simulink model "singlcontact_control_smc_lqr_mydimes_reaction"  (R2024a)
settings: Solver=VariableStepAuto  StartTime=0.0  StopTime=10  FixedStep=0.001  RelTol=1e-3
values from neighbouring files (symbols this model uses):
  ankle_servo_kd = 8    [robotParametersCtrl_mydiem_block_zmp.m]    (also in robotParametersCtrl_quad_modify_mydiem.m; robotParametersCtrl_quad_modify_mydiem_reaction.m)
  ankle_servo_ki = 4    [robotParametersCtrl_mydiem_block_zmp.m]    (also in robotParametersCtrl_quad_modify_mydiem.m; robotParametersCtrl_quad_modify_mydiem_reaction.m)
  ankle_servo_kp = 20    [robotParametersCtrl_mydiem_block_zmp.m]    (also in robotParametersCtrl_quad_modify_mydiem.m; robotParametersCtrl_quad_modify_mydiem_reaction.m)
  deriv_filter_coeff = 100    [robotParametersCtrl_mydiem_block_zmp.m]    (also in robotParametersCtrl_quad_modify_mydiem.m; robotParametersCtrl_quad_modify_mydiem_reaction.m)
  filter_coefficent_pid = 100    [robotParametersCtrl_mydiem_block_zmp.m]    (also in robotParametersCtrl_quad_modify_mydiem.m; robotParametersCtrl_quad_modify_mydiem_reaction.m)
  filter_coefficent_pids = 100    [robotParametersCtrl_quad_modify_mydiem_reaction.m]
  foot_z = 1.5    [robotParametersCtrl_mydiem_block_zmp.m]    (also in robotParametersCtrl_quad_modify_mydiem.m; robotParametersCtrl_quad_modify_mydiem_reaction.m)
  g = 9.81    [ABCDvalues_lqr_quad_mydime_reaction.m]    (also in robotParametersCtrl_mydiem_block_zmp.m = 9.80665; robotParametersCtrl_quad_modify_mydiem.m = 9.80665; robotParametersCtrl_quad_modify_mydiem_reaction.m = 9.80665)
  h = 32    [robotParametersCtrl_mydiem_block_zmp.m]    (also in robotParametersCtrl_quad_modify_mydiem.m; robotParametersCtrl_quad_modify_mydiem_reaction.m)
  height_plane = 0.025    [robotParametersCtrl_mydiem_block_zmp.m]    (also in robotParametersCtrl_quad_modify_mydiem.m; robotParametersCtrl_quad_modify_mydiem_reaction.m)
  hip_pitch_deriv = 20    [robotParametersCtrl_mydiem_block_zmp.m]    (also in robotParametersCtrl_quad_modify_mydiem.m = 200; robotParametersCtrl_quad_modify_mydiem_reaction.m = 200)
  hip_pitch_derivs = 200    [robotParametersCtrl_quad_modify_mydiem_reaction.m]
  hip_pitch_int = 0    [robotParametersCtrl_mydiem_block_zmp.m]    (also in robotParametersCtrl_quad_modify_mydiem.m = 150; robotParametersCtrl_quad_modify_mydiem_reaction.m = 150)
  hip_pitch_ints = 1500    [robotParametersCtrl_quad_modify_mydiem_reaction.m]
  hip_pitch_prop = 10    [robotParametersCtrl_mydiem_block_zmp.m]    (also in robotParametersCtrl_quad_modify_mydiem.m = 500; robotParametersCtrl_quad_modify_mydiem_reaction.m = 500)
  hip_pitch_props = 500    [robotParametersCtrl_quad_modify_mydiem_reaction.m]
  hip_roll_deriv = 28    [robotParametersCtrl_mydiem_block_zmp.m]    (also in robotParametersCtrl_quad_modify_mydiem.m = 280; robotParametersCtrl_quad_modify_mydiem_reaction.m = 280)
  hip_roll_derivs = 280    [robotParametersCtrl_quad_modify_mydiem_reaction.m]
  hip_roll_int = 0    [robotParametersCtrl_mydiem_block_zmp.m]    (also in robotParametersCtrl_quad_modify_mydiem.m = 180; robotParametersCtrl_quad_modify_mydiem_reaction.m = 180)
  hip_roll_ints = 180    [robotParametersCtrl_quad_modify_mydiem_reaction.m]
  hip_roll_prop = 10    [robotParametersCtrl_mydiem_block_zmp.m]    (also in robotParametersCtrl_quad_modify_mydiem.m = 300; robotParametersCtrl_quad_modify_mydiem_reaction.m = 300)
  hip_roll_props = 300    [robotParametersCtrl_quad_modify_mydiem_reaction.m]
  hip_servo_kd = 20    [robotParametersCtrl_mydiem_block_zmp.m]    (also in robotParametersCtrl_quad_modify_mydiem.m; robotParametersCtrl_quad_modify_mydiem_reaction.m)
  hip_servo_ki = 10    [robotParametersCtrl_mydiem_block_zmp.m]    (also in robotParametersCtrl_quad_modify_mydiem.m; robotParametersCtrl_quad_modify_mydiem_reaction.m)
  hip_servo_kp = 60    [robotParametersCtrl_mydiem_block_zmp.m]    (also in robotParametersCtrl_quad_modify_mydiem.m; robotParametersCtrl_quad_modify_mydiem_reaction.m)
  hip_smc_lamda = 85    [robotParametersCtrl_mydiem_block_zmp.m]    (also in robotParametersCtrl_quad_modify_mydiem.m; robotParametersCtrl_quad_modify_mydiem_reaction.m = 95)
  hip_smc_lamdas = 85    [robotParametersCtrl_quad_modify_mydiem_reaction.m]
  hip_smc_new = 25    [robotParametersCtrl_mydiem_block_zmp.m]    (also in robotParametersCtrl_quad_modify_mydiem.m; robotParametersCtrl_quad_modify_mydiem_reaction.m = 45)
  hip_smc_news = 25    [robotParametersCtrl_quad_modify_mydiem_reaction.m]
  init_angs_L = init_angs_R    [robotParametersCtrl_mydiem_block_zmp.m]    (also in robotParametersCtrl_quad_modify_mydiem.m; robotParametersCtrl_quad_modify_mydiem_reaction.m)
  init_angs_R = [0 -sum(init_angs) init_angs(2) 0 init_angs(1)]    [robotParametersCtrl_mydiem_block_zmp.m]    (also in robotParametersCtrl_quad_modify_mydiem.m; robotParametersCtrl_quad_modify_mydiem_reaction.m)
  init_height = h +                torso_z/2 + torso_offset_z + height_plane/2    (= 39.5125)    [robotParametersCtrl_mydiem_block_zmp.m]    (also in robotParametersCtrl_quad_modify_mydiem.m; robotParametersCtrl_quad_modify_mydiem_reaction.m)
  K = lqr(A, B, Q, R)    [ABCDvalues_lqr_quad_mydime_reaction.m]
  knee_pitch_deriv = 10    [robotParametersCtrl_mydiem_block_zmp.m]    (also in robotParametersCtrl_quad_modify_mydiem.m = 100; robotParametersCtrl_quad_modify_mydiem_reaction.m = 100)
  knee_pitch_derivs = 180    [robotParametersCtrl_quad_modify_mydiem_reaction.m]
  knee_pitch_int = 0    [robotParametersCtrl_mydiem_block_zmp.m]    (also in robotParametersCtrl_quad_modify_mydiem.m = 300; robotParametersCtrl_quad_modify_mydiem_reaction.m = 300)
  knee_pitch_ints = 7500    [robotParametersCtrl_quad_modify_mydiem_reaction.m]
  knee_pitch_prop = 10    [robotParametersCtrl_mydiem_block_zmp.m]    (also in robotParametersCtrl_quad_modify_mydiem.m = 400; robotParametersCtrl_quad_modify_mydiem_reaction.m = 400)
  knee_pitch_props = 1200    [robotParametersCtrl_quad_modify_mydiem_reaction.m]
  knee_servo_kd = 10    [robotParametersCtrl_mydiem_block_zmp.m]    (also in robotParametersCtrl_quad_modify_mydiem.m; robotParametersCtrl_quad_modify_mydiem_reaction.m)
  knee_servo_ki = 5    [robotParametersCtrl_mydiem_block_zmp.m]    (also in robotParametersCtrl_quad_modify_mydiem.m; robotParametersCtrl_quad_modify_mydiem_reaction.m)
  knee_servo_kp = 60    [robotParametersCtrl_mydiem_block_zmp.m]    (also in robotParametersCtrl_quad_modify_mydiem.m; robotParametersCtrl_quad_modify_mydiem_reaction.m)
  knee_smc_lamda = 140    [robotParametersCtrl_mydiem_block_zmp.m]    (also in robotParametersCtrl_quad_modify_mydiem.m; robotParametersCtrl_quad_modify_mydiem_reaction.m = 150)
  knee_smc_lamdas = 100    [robotParametersCtrl_quad_modify_mydiem_reaction.m]
  knee_smc_new = 80    [robotParametersCtrl_mydiem_block_zmp.m]    (also in robotParametersCtrl_quad_modify_mydiem.m; robotParametersCtrl_quad_modify_mydiem_reaction.m)
  knee_smc_news = 60    [robotParametersCtrl_quad_modify_mydiem_reaction.m]
  Kwalk = 0.6    [robotParametersCtrl_mydiem_block_zmp.m]    (also in robotParametersCtrl_quad_modify_mydiem.m; robotParametersCtrl_quad_modify_mydiem_reaction.m)
  l1 = 0.20    (= 0.2)    [ABCDvalues_lqr_quad_mydime_reaction.m]
  l2 = 0.20    (= 0.2)    [ABCDvalues_lqr_quad_mydime_reaction.m]
  lower_leg_length = 20    [robotParametersCtrl_mydiem_block_zmp.m]    (also in robotParametersCtrl_quad_modify_mydiem.m; robotParametersCtrl_quad_modify_mydiem_reaction.m)
  m1 = 0.45    [ABCDvalues_lqr_quad_mydime_reaction.m]
  m2 = 0.065    [ABCDvalues_lqr_quad_mydime_reaction.m]
  max_torque = 20    [robotParametersCtrl_mydiem_block_zmp.m]    (also in robotParametersCtrl_quad_modify_mydiem.m; robotParametersCtrl_quad_modify_mydiem_reaction.m)
  motion_time_constant = 0.01    [robotParametersCtrl_mydiem_block_zmp.m]    (also in robotParametersCtrl_quad_modify_mydiem.m; robotParametersCtrl_quad_modify_mydiem_reaction.m)
  plane_x = 25    [robotParametersCtrl_mydiem_block_zmp.m]    (also in robotParametersCtrl_quad_modify_mydiem.m; robotParametersCtrl_quad_modify_mydiem_reaction.m)
  plane_y = 3    [robotParametersCtrl_mydiem_block_zmp.m]    (also in robotParametersCtrl_quad_modify_mydiem.m; robotParametersCtrl_quad_modify_mydiem_reaction.m)
  stepHeight = 0.4    [ABCDvalues_lqr_quad_mydime_reaction.m]
  torso_offset_x = 17    [robotParametersCtrl_mydiem_block_zmp.m]    (also in robotParametersCtrl_quad_modify_mydiem.m; robotParametersCtrl_quad_modify_mydiem_reaction.m)
  torso_offset_x1 = -17    [robotParametersCtrl_mydiem_block_zmp.m]    (also in robotParametersCtrl_quad_modify_mydiem.m; robotParametersCtrl_quad_modify_mydiem_reaction.m)
  torso_offset_z = 0    [robotParametersCtrl_mydiem_block_zmp.m]    (also in robotParametersCtrl_quad_modify_mydiem.m; robotParametersCtrl_quad_modify_mydiem_reaction.m)
  torso_x = 40    [robotParametersCtrl_mydiem_block_zmp.m]    (also in robotParametersCtrl_quad_modify_mydiem.m; robotParametersCtrl_quad_modify_mydiem_reaction.m)
  torso_y = 20    [robotParametersCtrl_mydiem_block_zmp.m]    (also in robotParametersCtrl_quad_modify_mydiem.m; robotParametersCtrl_quad_modify_mydiem_reaction.m)
  torso_z = 15    [robotParametersCtrl_mydiem_block_zmp.m]    (also in robotParametersCtrl_quad_modify_mydiem.m; robotParametersCtrl_quad_modify_mydiem_reaction.m)
  Ts = 0.05    [ABCDvalues_lqr_quad_mydime_reaction.m]
  TsCtrl = 0.05    [robotParametersCtrl_mydiem_block_zmp.m]    (also in robotParametersCtrl_quad_modify_mydiem.m; robotParametersCtrl_quad_modify_mydiem_reaction.m)
  tWalk = 0.3    [robotParametersCtrl_mydiem_block_zmp.m]    (also in robotParametersCtrl_quad_modify_mydiem.m; robotParametersCtrl_quad_modify_mydiem_reaction.m)
  upper_leg_length = 20    [robotParametersCtrl_mydiem_block_zmp.m]    (also in robotParametersCtrl_quad_modify_mydiem.m; robotParametersCtrl_quad_modify_mydiem_reaction.m)
undefined symbols (not defined in the file or in its folder): X, Y, Z
libraries: simulink_extras x256, slpidlib x128, sm_lib x71, simulink x43, nesl_utility x35, walkingRobotUtils x21, dspsrcs4 x18, dspobslib x8
(part 23 of 33)

== system singlcontact_control_smc_lqr_mydimes_reaction/Walking Robot/smc+lqr/SMC Controllers FR2/SMC ==
  In1 : Inport
  In2 : Inport  Port=2
  T1_neuro : Inport  Port=3
  T2_neuro : Inport  Port=4
  Add : Sum
  Add1 : Sum
  Edot : Derivative
  Edot1 : Derivative
  Gain : Gain  Gain=-0.9
  Gain1 : Gain  Gain=-0.9
  Mux : Mux  Inputs=2
  New : Gain  Gain=knee_smc_new
  New1 : Gain  Gain=hip_smc_new
  Product : Product
  Product2 : Product
  S : Sum
  S1 : Sum
  Scope : Scope  NumInputPorts=2
  Scope{2..5} (4 alike) : Scope
  Sum : Sum  Inputs=++++
  Sum1 : Sum  Inputs=++++
  Tanh : Trigonometry  Operator=tanh
  Tanh1 : Trigonometry  Operator=tanh
  lamda : Constant  Value=knee_smc_lamda
  lamda1 : Constant  Value=hip_smc_lamda
  Out1 : Outport
  tag scope: edotBR1=global, edotBR2=global, lamdaBR1=global, lamdaBR2=global
  wires:
  S1/1 -> Tanh/1
  Edot/1 -> [edotBR1], S/1
  Product/1 -> S/2
  lamda1/1 -> [lamdaBR2], Product2/1
  In2/1 -> Product2/2, Edot1/1
  New1/1 -> Add1/1, Sum1/1
  Product2/1 -> S1/2
  In1/1 -> Edot/1, Product/2
  Edot1/1 -> S1/1, [edotBR2]
  Tanh1/1 -> New/1
  lamda/1 -> [lamdaBR1], Product/1
  Tanh/1 -> New1/1
  New/1 -> Sum/1, Add/1, Scope/1
  [TT1BR] -> Scope/2, Add/2, Sum/2
  [TT2BR] -> Add1/2, Sum1/2
  Mux/1 -> Out1/1
  Sum/1 -> Scope3/1, Scope5/1, Mux/1
  Sum1/1 -> Scope4/1, Mux/2, Scope2/1
  T1_neuro/1 -> Sum/3
  T2_neuro/1 -> Sum1/3
  S/1 -> Tanh1/1
  Add/1 -> Gain/1
  Gain/1 -> ?
  Gain1/1 -> ?
  Add1/1 -> Gain1/1

== system singlcontact_control_smc_lqr_mydimes_reaction/Walking Robot/smc+lqr/SMC Controllers FR3/Equivalent control ==
  theta2 : Inport
  theta1 : Inport  Port=2
  theta2ddot : Inport  Port=3
  theta1dot : Inport  Port=4
  theta2dot : Inport  Port=5
  theta1ddot : Inport  Port=6
  theta3 : Inport  Port=7
  theta4 : Inport  Port=8
  theta1dot1 : Inport  Port=9
  Constant : Constant  Value=0
  Constant1 : Constant  Value=0
  SMC equivalent T1 : Subsystem
  SMC equivalent T2 : Subsystem
  Scope : Scope  NumInputPorts=2
  tag scope: TT1BL=global, TT2BL=global
  wires:
  theta1dot1/1 -> SMC equivalent T2/5(theta1dot)
  theta2dot/1 -> SMC equivalent T1/5(theta2dot)
  theta1ddot/1 -> SMC equivalent T2/1(theta1ddot)
  theta4/1 -> SMC equivalent T2/3(theta1)
  theta1/1 -> SMC equivalent T1/2(theta1)
  theta3/1 -> SMC equivalent T2/2(theta2)
  Constant/1 -> SMC equivalent T1/6(theta1ddot)
  theta1dot/1 -> SMC equivalent T1/4(theta1dot)
  theta2ddot/1 -> SMC equivalent T1/3(theta2ddot)
  Constant1/1 -> SMC equivalent T2/4(theta2ddot)
  SMC equivalent T1/1(T1) -> [TT1BL], Scope/2
  theta2/1 -> SMC equivalent T1/1(theta2)
  SMC equivalent T2/1(T2) -> [TT2BL], Scope/1

== system singlcontact_control_smc_lqr_mydimes_reaction/Walking Robot/smc+lqr/SMC Controllers FR3/SMC ==
  In1 : Inport
  In2 : Inport  Port=2
  T1_neuro : Inport  Port=3
  T2_neuro : Inport  Port=4
  Add : Sum
  Add1 : Sum
  Edot : Derivative
  Edot1 : Derivative
  Gain : Gain  Gain=-0.9
  Gain1 : Gain  Gain=-0.9
  Mux : Mux  Inputs=2
  New : Gain  Gain=knee_smc_new
  New1 : Gain  Gain=hip_smc_new
  Product : Product
  Product2 : Product
  S : Sum
  S1 : Sum
  Scope : Scope  NumInputPorts=2
  Scope{2..5} (4 alike) : Scope
  Sum : Sum  Inputs=++++
  Sum1 : Sum  Inputs=++++
  Tanh : Trigonometry  Operator=tanh
  Tanh1 : Trigonometry  Operator=tanh
  lamda : Constant  Value=knee_smc_lamda
  lamda1 : Constant  Value=hip_smc_lamda
  Out1 : Outport
  tag scope: edotBL1=global, edotBL2=global, lamdaBL1=global, lamdaBL2=global
  wires:
  Add1/1 -> Gain1/1
  Gain1/1 -> ?
  Gain/1 -> ?
  Add/1 -> Gain/1
  S/1 -> Tanh1/1
  T2_neuro/1 -> Sum1/3
  T1_neuro/1 -> Sum/3
  Sum1/1 -> Scope2/1, Mux/2, Scope4/1
  Sum/1 -> Mux/1, Scope5/1, Scope3/1
  Mux/1 -> Out1/1
  [TT2BL] -> Sum1/2, Add1/2
  [TT1BL] -> Sum/2, Add/2, Scope/2
  New/1 -> Scope/1, Add/1, Sum/1
  Tanh/1 -> New1/1
  lamda/1 -> Product/1, [lamdaBL1]
  Tanh1/1 -> New/1
  Edot1/1 -> [edotBL2], S1/1
  In1/1 -> Product/2, Edot/1
  Product2/1 -> S1/2
  New1/1 -> Sum1/1, Add1/1
  In2/1 -> Edot1/1, Product2/2
  lamda1/1 -> Product2/1, [lamdaBL2]
  Product/1 -> S/2
  Edot/1 -> S/1, [edotBL1]
  S1/1 -> Tanh/1

== system singlcontact_control_smc_lqr_mydimes_reaction/Walking Robot/smc+lqr/SMC Controllers FR4/Equivalent control ==
  theta2 : Inport
  theta1 : Inport  Port=2
  theta2ddot : Inport  Port=3
  theta1dot : Inport  Port=4
  theta2dot : Inport  Port=5
  theta1ddot : Inport  Port=6
  theta3 : Inport  Port=7
  theta4 : Inport  Port=8
  theta1dot1 : Inport  Port=9
  Constant : Constant  Value=0
  Constant1 : Constant  Value=0
  SMC equivalent T1 : Subsystem
  SMC equivalent T2 : Subsystem
  Scope : Scope  NumInputPorts=2
  tag scope: TT1FR=global, TT2FR=global
  wires:
  SMC equivalent T2/1(T2) -> Scope/1, [TT2FR]
  theta2/1 -> SMC equivalent T1/1(theta2)
  SMC equivalent T1/1(T1) -> Scope/2, [TT1FR]
  Constant1/1 -> SMC equivalent T2/4(theta2ddot)
  theta2ddot/1 -> SMC equivalent T1/3(theta2ddot)
  theta1dot/1 -> SMC equivalent T1/4(theta1dot)
  Constant/1 -> SMC equivalent T1/6(theta1ddot)
  theta3/1 -> SMC equivalent T2/2(theta2)
  theta1/1 -> SMC equivalent T1/2(theta1)
  theta4/1 -> SMC equivalent T2/3(theta1)
  theta1ddot/1 -> SMC equivalent T2/1(theta1ddot)
  theta2dot/1 -> SMC equivalent T1/5(theta2dot)
  theta1dot1/1 -> SMC equivalent T2/5(theta1dot)

== system singlcontact_control_smc_lqr_mydimes_reaction/Walking Robot/smc+lqr/SMC Controllers FR4/SMC ==
  In1 : Inport
  In2 : Inport  Port=2
  T1_neuro : Inport  Port=3
  T2_neuro : Inport  Port=4
  Add : Sum
  Add1 : Sum
  Edot : Derivative
  Edot1 : Derivative
  Gain : Gain  Gain=-0.9
  Gain1 : Gain  Gain=-0.9
  Mux : Mux  Inputs=2
  New : Gain  Gain=knee_smc_new
  New1 : Gain  Gain=hip_smc_new
  Product : Product
  Product2 : Product
  S : Sum
  S1 : Sum
  Scope : Scope  NumInputPorts=2
  Scope{2..5} (4 alike) : Scope
  Sum : Sum  Inputs=++++
  Sum1 : Sum  Inputs=++++
  Tanh : Trigonometry  Operator=tanh
  Tanh1 : Trigonometry  Operator=tanh
  lamda : Constant  Value=knee_smc_lamda
  lamda1 : Constant  Value=hip_smc_lamda
  Out1 : Outport
  tag scope: edotFR1=global, edotFR2=global, lamdaFR1=global, lamdaFR2=global
  wires:
  S1/1 -> Tanh/1
  Edot/1 -> [edotFR1], S/1
  Product/1 -> S/2
  lamda1/1 -> [lamdaFR2], Product2/1
  In2/1 -> Product2/2, Edot1/1
  New1/1 -> Add1/1, Sum1/1
  Product2/1 -> S1/2
  In1/1 -> Edot/1, Product/2
  Edot1/1 -> S1/1, [edotFR2]
  Tanh1/1 -> New/1
  lamda/1 -> [lamdaFR1], Product/1
  Tanh/1 -> New1/1
  New/1 -> Sum/1, Add/1, Scope/1
  [TT1FR] -> Scope/2, Add/2, Sum/2
  [TT2FR] -> Add1/2, Sum1/2
  Mux/1 -> Out1/1
  Sum/1 -> Scope3/1, Scope5/1, Mux/1
  Sum1/1 -> Scope4/1, Mux/2, Scope2/1
  T1_neuro/1 -> Sum/3
  T2_neuro/1 -> Sum1/3
  S/1 -> Tanh1/1
  Add/1 -> Gain/1
  Gain/1 -> ?
  Gain1/1 -> ?
  Add1/1 -> Gain1/1

== system singlcontact_control_smc_lqr_mydimes_reaction/Walking Robot/smc+lqr+neuro1+reaction1/SMC Controllers BL/Equivalent control ==
  theta2 : Inport
  theta1 : Inport  Port=2
  theta2ddot : Inport  Port=3
  theta1dot : Inport  Port=4
  theta2dot : Inport  Port=5
  theta1ddot : Inport  Port=6
  theta3 : Inport  Port=7
  theta4 : Inport  Port=8
  theta1dot1 : Inport  Port=9
  Constant : Constant  Value=0
  Constant1 : Constant  Value=0
  SMC equivalent T1 : Subsystem
  SMC equivalent T2 : Subsystem
  Scope : Scope  NumInputPorts=2
  tag scope: TT1BL=global, TT2BL=global
  wires:
  theta1dot1/1 -> SMC equivalent T2/5(theta1dot)
  theta2dot/1 -> SMC equivalent T1/5(theta2dot)
  theta1ddot/1 -> SMC equivalent T2/1(theta1ddot)
  theta4/1 -> SMC equivalent T2/3(theta1)
  theta1/1 -> SMC equivalent T1/2(theta1)
  theta3/1 -> SMC equivalent T2/2(theta2)
  Constant/1 -> SMC equivalent T1/6(theta1ddot)
  theta1dot/1 -> SMC equivalent T1/4(theta1dot)
  theta2ddot/1 -> SMC equivalent T1/3(theta2ddot)
  Constant1/1 -> SMC equivalent T2/4(theta2ddot)
  SMC equivalent T1/1(T1) -> [TT1BL], Scope/2
  theta2/1 -> SMC equivalent T1/1(theta2)
  SMC equivalent T2/1(T2) -> [TT2BL], Scope/1

== system singlcontact_control_smc_lqr_mydimes_reaction/Walking Robot/smc+lqr+neuro1+reaction1/SMC Controllers BL/SMC ==
  In1 : Inport
  In2 : Inport  Port=2
  T1_neuro : Inport  Port=3
  T2_neuro : Inport  Port=4
  Input : Inport  Port=5
  Input1 : Inport  Port=6
  Edot : Derivative
  Edot1 : Derivative
  Gain : Gain  Gain=-0.85
  Gain1 : Gain  Gain=-0.7
  Mux : Mux  Inputs=2
  New : Gain  Gain=knee_smc_new
  New1 : Gain  Gain=hip_smc_new
  Product : Product
  Product2 : Product
  Random Source1 : dspobslib/Random Source  SrcType=Uniform  NormMethod=Ziggurat  CltLength=12  MinVal=-1  MaxVal=1  MeanVal=0  VarVal=1  RepMode=Not repeatable  rawSeed=1  IsInherit=off  SampMode=Discrete  SampTime=0.005  SampFrame=1  DataType=Double  OutComplex=Real  OutputFrames=off
  Random Source2 : dspobslib/Random Source  SrcType=Uniform  NormMethod=Ziggurat  CltLength=12  MinVal=-1  MaxVal=1  MeanVal=0  VarVal=1  RepMode=Not repeatable  rawSeed=1  IsInherit=off  SampMode=Discrete  SampTime=0.005  SampFrame=1  DataType=Double  OutComplex=Real  OutputFrames=off
  S : Sum
  S1 : Sum
  Scope : Scope  NumInputPorts=2
  Scope{2..5} (4 alike) : Scope
  Sum : Sum  Inputs=+++++
  Sum1 : Sum  Inputs=+++++
  Tanh : Trigonometry  Operator=tanh
  Tanh1 : Trigonometry  Operator=tanh
  lamda : Constant  Value=knee_smc_lamda
  lamda1 : Constant  Value=hip_smc_lamda
  Out1 : Outport
  tag scope: edotBL1=global, edotBL2=global, lamdaBL1=global, lamdaBL2=global, slBL1=global, slBL2=global
  wires:
  New1/1 -> Sum1/1, Gain1/1
  Gain1/1 -> Sum1/4
  Gain/1 -> Sum/4
  New/1 -> Sum/1, Gain/1
  S/1 -> Tanh1/1, [slBL1]
  T2_neuro/1 -> Sum1/3
  T1_neuro/1 -> Sum/3
  Sum1/1 -> Scope2/1, Mux/2, Scope4/1
  Sum/1 -> Mux/1, Scope5/1, Scope3/1
  Mux/1 -> Out1/1
  [TT2BL] -> Sum1/2
  [TT1BL] -> Sum/2
  Tanh/1 -> New1/1
  lamda/1 -> Product/1, [lamdaBL1]
  Tanh1/1 -> New/1
  Edot1/1 -> [edotBL2], S1/1
  In1/1 -> Product/2, Edot/1
  Product2/1 -> S1/2
  In2/1 -> Edot1/1, Product2/2
  lamda1/1 -> Product2/1, [lamdaBL2]
  Product/1 -> S/2
  Edot/1 -> S/1, [edotBL1]
  S1/1 -> Tanh/1, [slBL2]
  Random Source1/1 -> ?
  Random Source2/1 -> ?
  Input/1 -> Sum/5
  Input1/1 -> Sum1/5

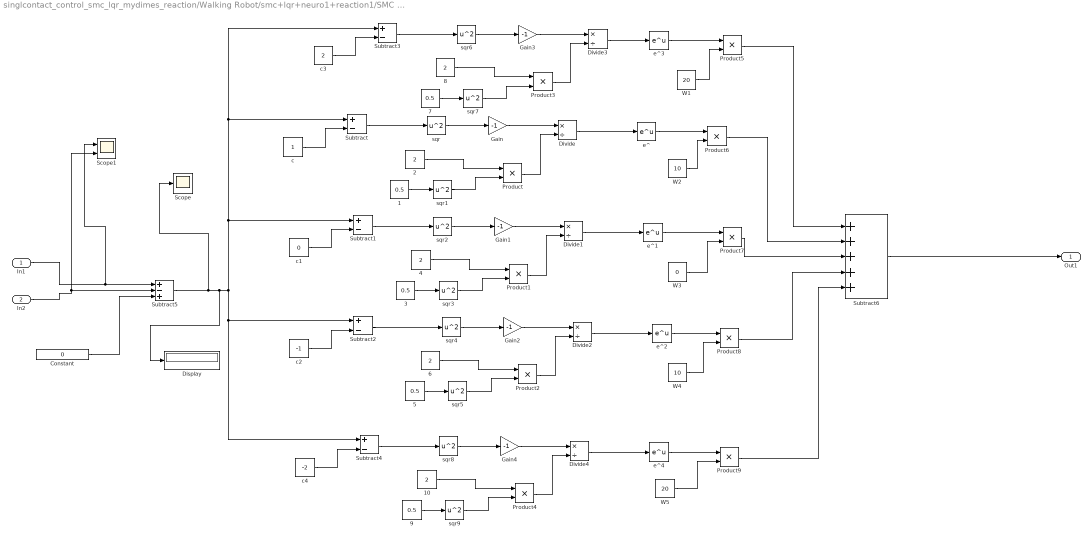
== system singlcontact_control_smc_lqr_mydimes_reaction/Walking Robot/smc+lqr+neuro1+reaction1/SMC Controllers BL/Subsystem ==
  In1 : Inport
  In2 : Inport  Port=2
  {1,3,5,7,9} (5 alike) : Constant  Value=0.5
  {2,4,6,8,10} (5 alike) : Constant  Value=2
  Constant : Constant  Value=0
  Display : Display
  Divide{,1..4} (5 alike) : Product  Inputs=*/
  Gain{,1..4} (5 alike) : Gain  Gain=-1
  Product{,1..9} (10 alike) : Product
  Scope : Scope
  Scope1 : Scope  NumInputPorts=2
  Subtract{,1..4} (5 alike) : Sum  Inputs=+-
  Subtract5 : Sum  Inputs=+-+
  Subtract6 : Sum  Inputs=+++++
  W1 : Constant  Value=20
  W2 : Constant  Value=10
  W3 : Constant  Value=0
  W4 : Constant  Value=10
  W5 : Constant  Value=20
  c : Constant
  c1 : Constant  Value=0
  c2 : Constant  Value=-1
  c3 : Constant  Value=2
  c4 : Constant  Value=-2
  e^{,1..4} (5 alike) : Math
  sqr{,1..9} (10 alike) : Math  Operator=square
  Out1 : Outport
  wires:
  Constant/1 -> Subtract5/3
  Divide3/1 -> e^3/1
  9/1 -> sqr9/1
  Product8/1 -> Subtract6/4
  Product7/1 -> Subtract6/3
  W4/1 -> Product8/2
  c2/1 -> Subtract2/2
  Product4/1 -> Divide4/2
  10/1 -> Product4/1
  e^3/1 -> Product5/1
  sqr6/1 -> Gain3/1
  6/1 -> Product2/1
  sqr3/1 -> Product1/2
  e^2/1 -> Product8/1
  Divide2/1 -> e^2/1
  Subtract2/1 -> sqr4/1
  Subtract6/1 -> Out1/1
  8/1 -> Product3/1
  sqr7/1 -> Product3/2
  Divide/1 -> e^/1
  5/1 -> sqr5/1
  3/1 -> sqr3/1
  4/1 -> Product1/1
  Gain2/1 -> Divide2/1
  Gain4/1 -> Divide4/1
  In1/1 -> Subtract5/1, Scope1/1
  W1/1 -> Product5/2
  sqr4/1 -> Gain2/1
  c3/1 -> Subtract3/2
  e^4/1 -> Product9/1
  sqr5/1 -> Product2/2
  sqr8/1 -> Gain4/1
  1/1 -> sqr1/1
  2/1 -> Product/1
  Product5/1 -> Subtract6/1
  Divide4/1 -> e^4/1
  W5/1 -> Product9/2
  7/1 -> sqr7/1
  Subtract/1 -> sqr/1
  Subtract5/1 -> Subtract2/1, Subtract4/1, Subtract3/1, Subtract/1, Subtract1/1, Display/1, Scope/1
  c1/1 -> Subtract1/2
  Subtract1/1 -> sqr2/1
  e^1/1 -> Product7/1
  Product9/1 -> Subtract6/5
  c4/1 -> Subtract4/2
  Subtract3/1 -> sqr6/1
  e^/1 -> Product6/1
  Product3/1 -> Divide3/2
  W2/1 -> Product6/2
  W3/1 -> Product7/2
  Gain1/1 -> Divide1/1
  Product6/1 -> Subtract6/2
  Product2/1 -> Divide2/2
  Gain/1 -> Divide/1
  Subtract4/1 -> sqr8/1
  Divide1/1 -> e^1/1
  Gain3/1 -> Divide3/1
  In2/1 -> Scope1/2, Subtract5/2
  sqr1/1 -> Product/2
  sqr2/1 -> Gain1/1
  Product/1 -> Divide/2
  sqr/1 -> Gain/1
  Product1/1 -> Divide1/2
  sqr9/1 -> Product4/2
  c/1 -> Subtract/2

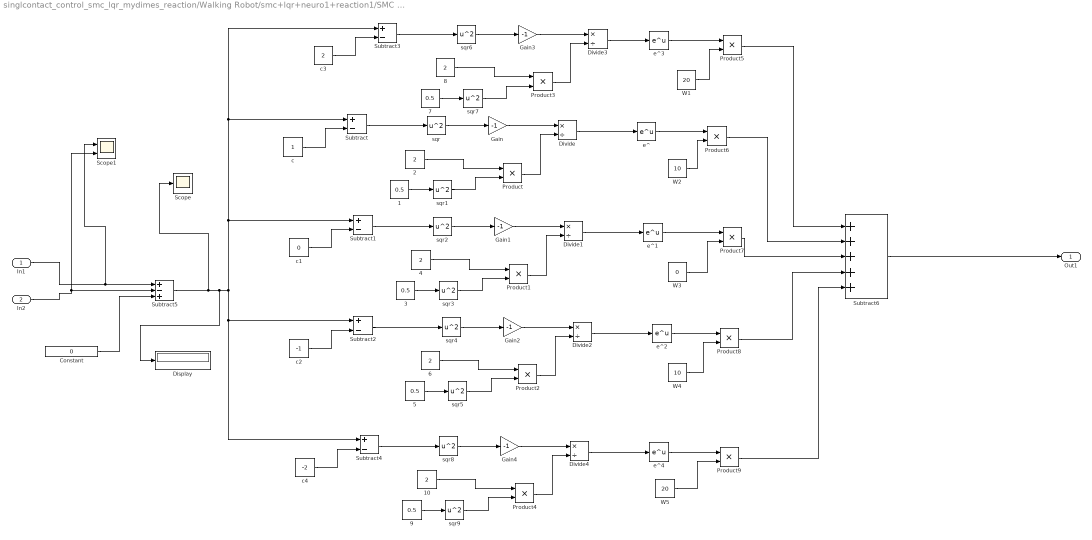
== system singlcontact_control_smc_lqr_mydimes_reaction/Walking Robot/smc+lqr+neuro1+reaction1/SMC Controllers BL/Subsystem1 ==
  In1 : Inport
  In2 : Inport  Port=2
  {1,3,5,7,9} (5 alike) : Constant  Value=0.5
  {2,4,6,8,10} (5 alike) : Constant  Value=2
  Constant : Constant  Value=0
  Display : Display
  Divide{,1..4} (5 alike) : Product  Inputs=*/
  Gain{,1..4} (5 alike) : Gain  Gain=-1
  Product{,1..9} (10 alike) : Product
  Scope : Scope
  Scope1 : Scope  NumInputPorts=2
  Subtract{,1..4} (5 alike) : Sum  Inputs=+-
  Subtract5 : Sum  Inputs=+-+
  Subtract6 : Sum  Inputs=+++++
  W1 : Constant  Value=20
  W2 : Constant  Value=10
  W3 : Constant  Value=0
  W4 : Constant  Value=10
  W5 : Constant  Value=20
  c : Constant
  c1 : Constant  Value=0
  c2 : Constant  Value=-1
  c3 : Constant  Value=2
  c4 : Constant  Value=-2
  e^{,1..4} (5 alike) : Math
  sqr{,1..9} (10 alike) : Math  Operator=square
  Out1 : Outport
  wires:
  c/1 -> Subtract/2
  sqr9/1 -> Product4/2
  Product1/1 -> Divide1/2
  sqr/1 -> Gain/1
  Product/1 -> Divide/2
  sqr2/1 -> Gain1/1
  sqr1/1 -> Product/2
  In2/1 -> Subtract5/2, Scope1/2
  Gain3/1 -> Divide3/1
  Divide1/1 -> e^1/1
  Subtract4/1 -> sqr8/1
  Gain/1 -> Divide/1
  Product2/1 -> Divide2/2
  Product6/1 -> Subtract6/2
  Gain1/1 -> Divide1/1
  W3/1 -> Product7/2
  W2/1 -> Product6/2
  Product3/1 -> Divide3/2
  e^/1 -> Product6/1
  Subtract3/1 -> sqr6/1
  c4/1 -> Subtract4/2
  Product9/1 -> Subtract6/5
  e^1/1 -> Product7/1
  Subtract1/1 -> sqr2/1
  c1/1 -> Subtract1/2
  Subtract5/1 -> Scope/1, Display/1, Subtract1/1, Subtract/1, Subtract3/1, Subtract4/1, Subtract2/1
  Subtract/1 -> sqr/1
  7/1 -> sqr7/1
  W5/1 -> Product9/2
  Divide4/1 -> e^4/1
  Product5/1 -> Subtract6/1
  2/1 -> Product/1
  1/1 -> sqr1/1
  sqr8/1 -> Gain4/1
  sqr5/1 -> Product2/2
  e^4/1 -> Product9/1
  c3/1 -> Subtract3/2
  sqr4/1 -> Gain2/1
  W1/1 -> Product5/2
  In1/1 -> Scope1/1, Subtract5/1
  Gain4/1 -> Divide4/1
  Gain2/1 -> Divide2/1
  4/1 -> Product1/1
  3/1 -> sqr3/1
  5/1 -> sqr5/1
  Divide/1 -> e^/1
  sqr7/1 -> Product3/2
  8/1 -> Product3/1
  Subtract6/1 -> Out1/1
  Subtract2/1 -> sqr4/1
  Divide2/1 -> e^2/1
  e^2/1 -> Product8/1
  sqr3/1 -> Product1/2
  6/1 -> Product2/1
  sqr6/1 -> Gain3/1
  e^3/1 -> Product5/1
  10/1 -> Product4/1
  Product4/1 -> Divide4/2
  c2/1 -> Subtract2/2
  W4/1 -> Product8/2
  Product7/1 -> Subtract6/3
  Product8/1 -> Subtract6/4
  9/1 -> sqr9/1
  Divide3/1 -> e^3/1
  Constant/1 -> Subtract5/3

== system singlcontact_control_smc_lqr_mydimes_reaction/Walking Robot/smc+lqr+neuro1+reaction1/SMC Controllers BL/Subsystem2 ==
  <knee_angle> : Inport
  <hip_pitch_angle> : Inport  Port=2
  Gain3 : Gain  Gain=0.5
  Product : Product
  Product3 : Product
  length from ground : Subsystem
  Input : Outport
  Input1 : Outport  Port=2
  wires:
  Product/1 -> Input/1
  length from ground/2(Outport) -> Product3/1
  Gain3/1 -> Product/2, Product3/2
  Product3/1 -> Input1/1
  [Rbl] -> Gain3/1
  <hip_pitch_angle>/1 -> length from ground/2(In2)
  <knee_angle>/1 -> length from ground/1(In1)
  length from ground/1(Output) -> Product/1

== system singlcontact_control_smc_lqr_mydimes_reaction/Walking Robot/smc+lqr+neuro1+reaction1/SMC Controllers BR/Equivalent control ==
  theta2 : Inport
  theta1 : Inport  Port=2
  theta2ddot : Inport  Port=3
  theta1dot : Inport  Port=4
  theta2dot : Inport  Port=5
  theta1ddot : Inport  Port=6
  theta3 : Inport  Port=7
  theta4 : Inport  Port=8
  theta1dot1 : Inport  Port=9
  Constant : Constant  Value=0
  Constant1 : Constant  Value=0
  SMC equivalent T1 : Subsystem
  SMC equivalent T2 : Subsystem
  Scope : Scope  NumInputPorts=2
  tag scope: TT1BR=global, TT2BR=global
  wires:
  SMC equivalent T2/1(T2) -> Scope/1, [TT2BR]
  theta2/1 -> SMC equivalent T1/1(theta2)
  SMC equivalent T1/1(T1) -> Scope/2, [TT1BR]
  Constant1/1 -> SMC equivalent T2/4(theta2ddot)
  theta2ddot/1 -> SMC equivalent T1/3(theta2ddot)
  theta1dot/1 -> SMC equivalent T1/4(theta1dot)
  Constant/1 -> SMC equivalent T1/6(theta1ddot)
  theta3/1 -> SMC equivalent T2/2(theta2)
  theta1/1 -> SMC equivalent T1/2(theta1)
  theta4/1 -> SMC equivalent T2/3(theta1)
  theta1ddot/1 -> SMC equivalent T2/1(theta1ddot)
  theta2dot/1 -> SMC equivalent T1/5(theta2dot)
  theta1dot1/1 -> SMC equivalent T2/5(theta1dot)

== system singlcontact_control_smc_lqr_mydimes_reaction/Walking Robot/smc+lqr+neuro1+reaction1/SMC Controllers BR/SMC ==
  In1 : Inport
  In2 : Inport  Port=2
  T1_neuro : Inport  Port=3
  T2_neuro : Inport  Port=4
  Input : Inport  Port=5
  Input1 : Inport  Port=6
  Edot : Derivative
  Edot1 : Derivative
  Gain : Gain  Gain=-0.85
  Gain1 : Gain  Gain=-0.7
  Mux : Mux  Inputs=2
  New : Gain  Gain=knee_smc_new
  New1 : Gain  Gain=hip_smc_new
  Product : Product
  Product2 : Product
  Random Source1 : dspobslib/Random Source  SrcType=Uniform  NormMethod=Ziggurat  CltLength=12  MinVal=-1  MaxVal=1  MeanVal=0  VarVal=1  RepMode=Not repeatable  rawSeed=1  IsInherit=off  SampMode=Discrete  SampTime=0.005  SampFrame=1  DataType=Double  OutComplex=Real  OutputFrames=off
  Random Source2 : dspobslib/Random Source  SrcType=Uniform  NormMethod=Ziggurat  CltLength=12  MinVal=-1  MaxVal=1  MeanVal=0  VarVal=1  RepMode=Not repeatable  rawSeed=1  IsInherit=off  SampMode=Discrete  SampTime=0.005  SampFrame=1  DataType=Double  OutComplex=Real  OutputFrames=off
  S : Sum
  S1 : Sum
  Scope : Scope  NumInputPorts=2
  Scope{2..5} (4 alike) : Scope
  Sum : Sum  Inputs=+++++
  Sum1 : Sum  Inputs=+++++
  Tanh : Trigonometry  Operator=tanh
  Tanh1 : Trigonometry  Operator=tanh
  lamda : Constant  Value=knee_smc_lamda
  lamda1 : Constant  Value=hip_smc_lamda
  Out1 : Outport
  tag scope: edotBR1=global, edotBR2=global, lamdaBR1=global, lamdaBR2=global, slBR1=global, slBR2=global
  wires:
  S1/1 -> [slBR2], Tanh/1
  Edot/1 -> [edotBR1], S/1
  Product/1 -> S/2
  lamda1/1 -> Product2/1, [lamdaBR2]
  In2/1 -> Product2/2, Edot1/1
  Product2/1 -> S1/2
  In1/1 -> Edot/1, Product/2
  Edot1/1 -> S1/1, [edotBR2]
  Tanh1/1 -> New/1
  lamda/1 -> [lamdaBR1], Product/1
  Tanh/1 -> New1/1
  [TT1BR] -> Sum/2
  [TT2BR] -> Sum1/2
  Mux/1 -> Out1/1
  Sum/1 -> Mux/1, Scope5/1, Scope3/1
  Sum1/1 -> Scope4/1, Mux/2, Scope2/1
  T1_neuro/1 -> Sum/3
  T2_neuro/1 -> Sum1/3
  S/1 -> [slBR1], Tanh1/1
  New/1 -> Gain/1, Sum/1
  Gain/1 -> Sum/4
  Gain1/1 -> Sum1/4
  New1/1 -> Sum1/1, Gain1/1
  Random Source1/1 -> ?
  Random Source2/1 -> ?
  Input/1 -> Sum/5
  Input1/1 -> Sum1/5

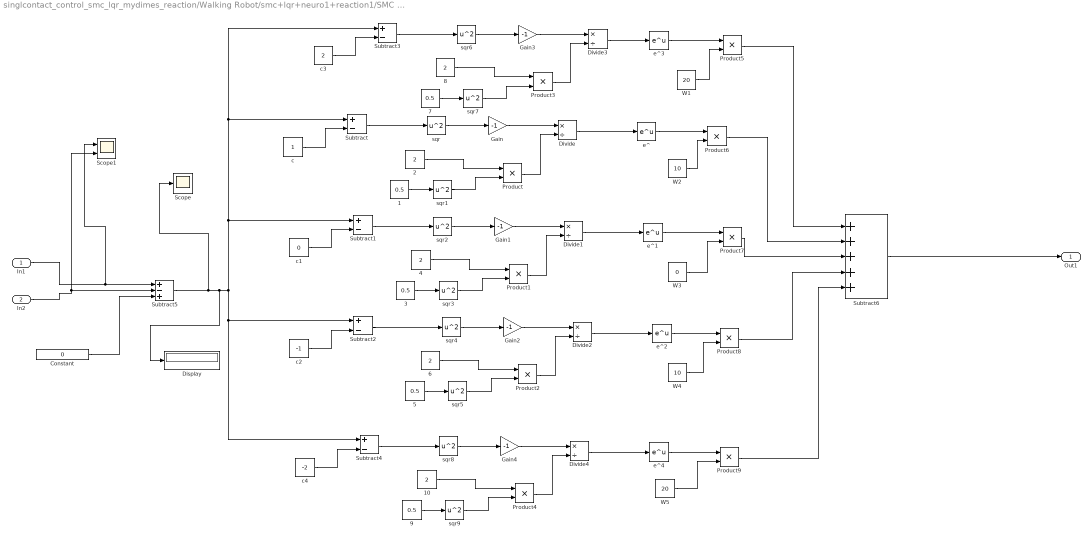
== system singlcontact_control_smc_lqr_mydimes_reaction/Walking Robot/smc+lqr+neuro1+reaction1/SMC Controllers BR/Subsystem ==
  In1 : Inport
  In2 : Inport  Port=2
  {1,3,5,7,9} (5 alike) : Constant  Value=0.5
  {2,4,6,8,10} (5 alike) : Constant  Value=2
  Constant : Constant  Value=0
  Display : Display
  Divide{,1..4} (5 alike) : Product  Inputs=*/
  Gain{,1..4} (5 alike) : Gain  Gain=-1
  Product{,1..9} (10 alike) : Product
  Scope : Scope
  Scope1 : Scope  NumInputPorts=2
  Subtract{,1..4} (5 alike) : Sum  Inputs=+-
  Subtract5 : Sum  Inputs=+-+
  Subtract6 : Sum  Inputs=+++++
  W1 : Constant  Value=20
  W2 : Constant  Value=10
  W3 : Constant  Value=0
  W4 : Constant  Value=10
  W5 : Constant  Value=20
  c : Constant
  c1 : Constant  Value=0
  c2 : Constant  Value=-1
  c3 : Constant  Value=2
  c4 : Constant  Value=-2
  e^{,1..4} (5 alike) : Math
  sqr{,1..9} (10 alike) : Math  Operator=square
  Out1 : Outport
  wires:
  c/1 -> Subtract/2
  sqr9/1 -> Product4/2
  Product1/1 -> Divide1/2
  sqr/1 -> Gain/1
  Product/1 -> Divide/2
  sqr2/1 -> Gain1/1
  sqr1/1 -> Product/2
  In2/1 -> Subtract5/2, Scope1/2
  Gain3/1 -> Divide3/1
  Divide1/1 -> e^1/1
  Subtract4/1 -> sqr8/1
  Gain/1 -> Divide/1
  Product2/1 -> Divide2/2
  Product6/1 -> Subtract6/2
  Gain1/1 -> Divide1/1
  W3/1 -> Product7/2
  W2/1 -> Product6/2
  Product3/1 -> Divide3/2
  e^/1 -> Product6/1
  Subtract3/1 -> sqr6/1
  c4/1 -> Subtract4/2
  Product9/1 -> Subtract6/5
  e^1/1 -> Product7/1
  Subtract1/1 -> sqr2/1
  c1/1 -> Subtract1/2
  Subtract5/1 -> Scope/1, Display/1, Subtract1/1, Subtract/1, Subtract3/1, Subtract4/1, Subtract2/1
  Subtract/1 -> sqr/1
  7/1 -> sqr7/1
  W5/1 -> Product9/2
  Divide4/1 -> e^4/1
  Product5/1 -> Subtract6/1
  2/1 -> Product/1
  1/1 -> sqr1/1
  sqr8/1 -> Gain4/1
  sqr5/1 -> Product2/2
  e^4/1 -> Product9/1
  c3/1 -> Subtract3/2
  sqr4/1 -> Gain2/1
  W1/1 -> Product5/2
  In1/1 -> Scope1/1, Subtract5/1
  Gain4/1 -> Divide4/1
  Gain2/1 -> Divide2/1
  4/1 -> Product1/1
  3/1 -> sqr3/1
  5/1 -> sqr5/1
  Divide/1 -> e^/1
  sqr7/1 -> Product3/2
  8/1 -> Product3/1
  Subtract6/1 -> Out1/1
  Subtract2/1 -> sqr4/1
  Divide2/1 -> e^2/1
  e^2/1 -> Product8/1
  sqr3/1 -> Product1/2
  6/1 -> Product2/1
  sqr6/1 -> Gain3/1
  e^3/1 -> Product5/1
  10/1 -> Product4/1
  Product4/1 -> Divide4/2
  c2/1 -> Subtract2/2
  W4/1 -> Product8/2
  Product7/1 -> Subtract6/3
  Product8/1 -> Subtract6/4
  9/1 -> sqr9/1
  Divide3/1 -> e^3/1
  Constant/1 -> Subtract5/3

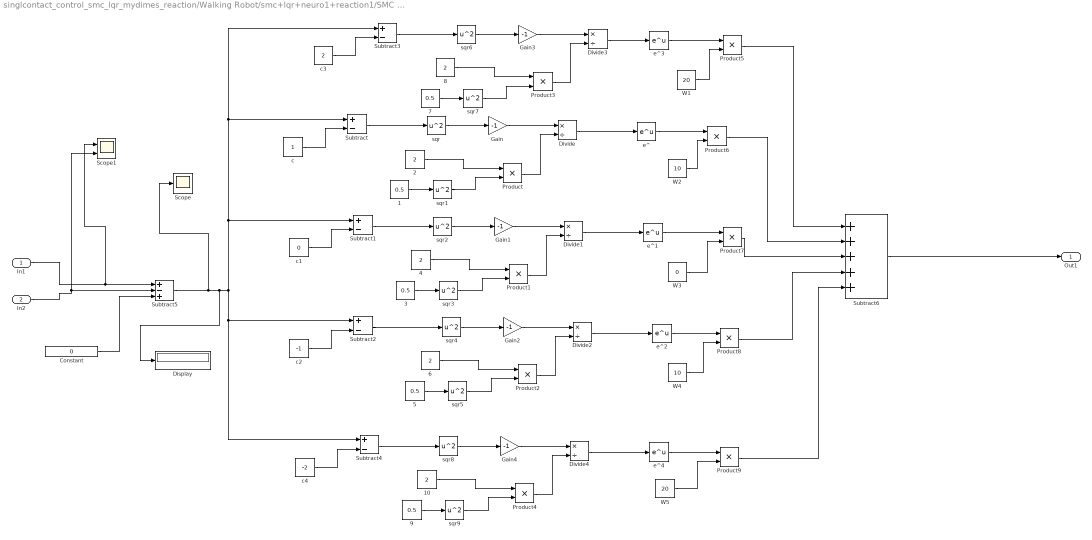
== system singlcontact_control_smc_lqr_mydimes_reaction/Walking Robot/smc+lqr+neuro1+reaction1/SMC Controllers BR/Subsystem1 ==
  In1 : Inport
  In2 : Inport  Port=2
  {1,3,5,7,9} (5 alike) : Constant  Value=0.5
  {2,4,6,8,10} (5 alike) : Constant  Value=2
  Constant : Constant  Value=0
  Display : Display
  Divide{,1..4} (5 alike) : Product  Inputs=*/
  Gain{,1..4} (5 alike) : Gain  Gain=-1
  Product{,1..9} (10 alike) : Product
  Scope : Scope
  Scope1 : Scope  NumInputPorts=2
  Subtract{,1..4} (5 alike) : Sum  Inputs=+-
  Subtract5 : Sum  Inputs=+-+
  Subtract6 : Sum  Inputs=+++++
  W1 : Constant  Value=20
  W2 : Constant  Value=10
  W3 : Constant  Value=0
  W4 : Constant  Value=10
  W5 : Constant  Value=20
  c : Constant
  c1 : Constant  Value=0
  c2 : Constant  Value=-1
  c3 : Constant  Value=2
  c4 : Constant  Value=-2
  e^{,1..4} (5 alike) : Math
  sqr{,1..9} (10 alike) : Math  Operator=square
  Out1 : Outport
  wires:
  Constant/1 -> Subtract5/3
  Divide3/1 -> e^3/1
  9/1 -> sqr9/1
  Product8/1 -> Subtract6/4
  Product7/1 -> Subtract6/3
  W4/1 -> Product8/2
  c2/1 -> Subtract2/2
  Product4/1 -> Divide4/2
  10/1 -> Product4/1
  e^3/1 -> Product5/1
  sqr6/1 -> Gain3/1
  6/1 -> Product2/1
  sqr3/1 -> Product1/2
  e^2/1 -> Product8/1
  Divide2/1 -> e^2/1
  Subtract2/1 -> sqr4/1
  Subtract6/1 -> Out1/1
  8/1 -> Product3/1
  sqr7/1 -> Product3/2
  Divide/1 -> e^/1
  5/1 -> sqr5/1
  3/1 -> sqr3/1
  4/1 -> Product1/1
  Gain2/1 -> Divide2/1
  Gain4/1 -> Divide4/1
  In1/1 -> Subtract5/1, Scope1/1
  W1/1 -> Product5/2
  sqr4/1 -> Gain2/1
  c3/1 -> Subtract3/2
  e^4/1 -> Product9/1
  sqr5/1 -> Product2/2
  sqr8/1 -> Gain4/1
  1/1 -> sqr1/1
  2/1 -> Product/1
  Product5/1 -> Subtract6/1
  Divide4/1 -> e^4/1
  W5/1 -> Product9/2
  7/1 -> sqr7/1
  Subtract/1 -> sqr/1
  Subtract5/1 -> Subtract2/1, Subtract4/1, Subtract3/1, Subtract/1, Subtract1/1, Display/1, Scope/1
  c1/1 -> Subtract1/2
  Subtract1/1 -> sqr2/1
  e^1/1 -> Product7/1
  Product9/1 -> Subtract6/5
  c4/1 -> Subtract4/2
  Subtract3/1 -> sqr6/1
  e^/1 -> Product6/1
  Product3/1 -> Divide3/2
  W2/1 -> Product6/2
  W3/1 -> Product7/2
  Gain1/1 -> Divide1/1
  Product6/1 -> Subtract6/2
  Product2/1 -> Divide2/2
  Gain/1 -> Divide/1
  Subtract4/1 -> sqr8/1
  Divide1/1 -> e^1/1
  Gain3/1 -> Divide3/1
  In2/1 -> Scope1/2, Subtract5/2
  sqr1/1 -> Product/2
  sqr2/1 -> Gain1/1
  Product/1 -> Divide/2
  sqr/1 -> Gain/1
  Product1/1 -> Divide1/2
  sqr9/1 -> Product4/2
  c/1 -> Subtract/2

== system singlcontact_control_smc_lqr_mydimes_reaction/Walking Robot/smc+lqr+neuro1+reaction1/SMC Controllers BR/Subsystem2 ==
  <knee_angle> : Inport
  <hip_pitch_angle> : Inport  Port=2
  Gain3 : Gain  Gain=0.5
  Product : Product
  Product3 : Product
  length from ground : Subsystem
  Input : Outport
  Input1 : Outport  Port=2
  wires:
  Product/1 -> Input/1
  length from ground/2(Outport) -> Product3/1
  Gain3/1 -> Product/2, Product3/2
  Product3/1 -> Input1/1
  [Rbr] -> Gain3/1
  <hip_pitch_angle>/1 -> length from ground/2(In2)
  <knee_angle>/1 -> length from ground/1(In1)
  length from ground/1(Output) -> Product/1

== system singlcontact_control_smc_lqr_mydimes_reaction/Walking Robot/smc+lqr+neuro1+reaction1/SMC Controllers FL/Equivalent control ==
  theta2 : Inport
  theta1 : Inport  Port=2
  theta2ddot : Inport  Port=3
  theta1dot : Inport  Port=4
  theta2dot : Inport  Port=5
  theta1ddot : Inport  Port=6
  theta3 : Inport  Port=7
  theta4 : Inport  Port=8
  theta1dot1 : Inport  Port=9
  Constant : Constant  Value=0
  Constant1 : Constant  Value=0
  SMC equivalent T1 : Subsystem
  SMC equivalent T2 : Subsystem
  Scope : Scope  NumInputPorts=2
  tag scope: TT1FL=global, TT2FL=global
  wires:
  theta1dot1/1 -> SMC equivalent T2/5(theta1dot)
  theta2dot/1 -> SMC equivalent T1/5(theta2dot)
  theta1ddot/1 -> SMC equivalent T2/1(theta1ddot)
  theta4/1 -> SMC equivalent T2/3(theta1)
  theta1/1 -> SMC equivalent T1/2(theta1)
  theta3/1 -> SMC equivalent T2/2(theta2)
  Constant/1 -> SMC equivalent T1/6(theta1ddot)
  theta1dot/1 -> SMC equivalent T1/4(theta1dot)
  theta2ddot/1 -> SMC equivalent T1/3(theta2ddot)
  Constant1/1 -> SMC equivalent T2/4(theta2ddot)
  SMC equivalent T1/1(T1) -> [TT1FL], Scope/2
  theta2/1 -> SMC equivalent T1/1(theta2)
  SMC equivalent T2/1(T2) -> [TT2FL], Scope/1

== system singlcontact_control_smc_lqr_mydimes_reaction/Walking Robot/smc+lqr+neuro1+reaction1/SMC Controllers FL/SMC ==
  In1 : Inport
  In2 : Inport  Port=2
  T1_neuro : Inport  Port=3
  T2_neuro : Inport  Port=4
  Input : Inport  Port=5
  Input1 : Inport  Port=6
  Edot : Derivative
  Edot1 : Derivative
  Gain : Gain  Gain=-0.85
  Gain1 : Gain  Gain=-0.7
  Mux : Mux  Inputs=2
  New : Gain  Gain=knee_smc_new
  New1 : Gain  Gain=hip_smc_new
  Product : Product
  Product2 : Product
  Random Source1 : dspobslib/Random Source  SrcType=Uniform  NormMethod=Ziggurat  CltLength=12  MinVal=-1  MaxVal=1  MeanVal=0  VarVal=1  RepMode=Not repeatable  rawSeed=1  IsInherit=off  SampMode=Discrete  SampTime=0.005  SampFrame=1  DataType=Double  OutComplex=Real  OutputFrames=off
  Random Source2 : dspobslib/Random Source  SrcType=Uniform  NormMethod=Ziggurat  CltLength=12  MinVal=-1  MaxVal=1  MeanVal=0  VarVal=1  RepMode=Not repeatable  rawSeed=1  IsInherit=off  SampMode=Discrete  SampTime=0.005  SampFrame=1  DataType=Double  OutComplex=Real  OutputFrames=off
  S : Sum
  S1 : Sum
  Scope : Scope  NumInputPorts=2
  Scope{2..5} (4 alike) : Scope
  Sum : Sum  Inputs=+++++
  Sum1 : Sum  Inputs=+++++
  Tanh : Trigonometry  Operator=tanh
  Tanh1 : Trigonometry  Operator=tanh
  lamda : Constant  Value=knee_smc_lamda
  lamda1 : Constant  Value=hip_smc_lamda
  Out1 : Outport
  tag scope: edotFL1=global, edotFL2=global, lamdaFL1=global, lamdaFL2=global, slFL1=global, slFL2=global
  wires:
  New1/1 -> Sum1/1, Gain1/1
  Gain1/1 -> Sum1/4
  Gain/1 -> Sum/4
  New/1 -> Sum/1, Gain/1
  S/1 -> Tanh1/1, [slFL1]
  T2_neuro/1 -> Sum1/3
  T1_neuro/1 -> Sum/3
  Sum1/1 -> Scope2/1, Mux/2, Scope4/1
  Sum/1 -> Mux/1, Scope5/1, Scope3/1
  Mux/1 -> Out1/1
  [TT2FL] -> Sum1/2
  [TT1FL] -> Sum/2
  Tanh/1 -> New1/1
  lamda/1 -> Product/1, [lamdaFL1]
  Tanh1/1 -> New/1
  Edot1/1 -> [edotFL2], S1/1
  In1/1 -> Product/2, Edot/1
  Product2/1 -> S1/2
  In2/1 -> Edot1/1, Product2/2
  lamda1/1 -> Product2/1, [lamdaFL2]
  Product/1 -> S/2
  Edot/1 -> S/1, [edotFL1]
  S1/1 -> Tanh/1, [slFL2]
  Random Source1/1 -> ?
  Random Source2/1 -> ?
  Input/1 -> Sum/5
  Input1/1 -> Sum1/5

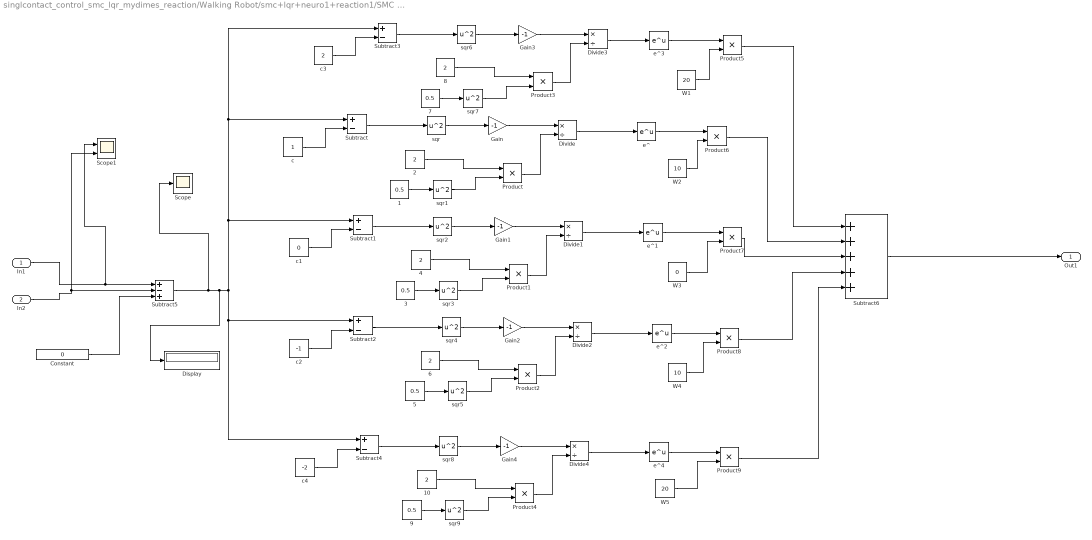
== system singlcontact_control_smc_lqr_mydimes_reaction/Walking Robot/smc+lqr+neuro1+reaction1/SMC Controllers FL/Subsystem ==
  In1 : Inport
  In2 : Inport  Port=2
  {1,3,5,7,9} (5 alike) : Constant  Value=0.5
  {2,4,6,8,10} (5 alike) : Constant  Value=2
  Constant : Constant  Value=0
  Display : Display
  Divide{,1..4} (5 alike) : Product  Inputs=*/
  Gain{,1..4} (5 alike) : Gain  Gain=-1
  Product{,1..9} (10 alike) : Product
  Scope : Scope
  Scope1 : Scope  NumInputPorts=2
  Subtract{,1..4} (5 alike) : Sum  Inputs=+-
  Subtract5 : Sum  Inputs=+-+
  Subtract6 : Sum  Inputs=+++++
  W1 : Constant  Value=20
  W2 : Constant  Value=10
  W3 : Constant  Value=0
  W4 : Constant  Value=10
  W5 : Constant  Value=20
  c : Constant
  c1 : Constant  Value=0
  c2 : Constant  Value=-1
  c3 : Constant  Value=2
  c4 : Constant  Value=-2
  e^{,1..4} (5 alike) : Math
  sqr{,1..9} (10 alike) : Math  Operator=square
  Out1 : Outport
  wires:
  Constant/1 -> Subtract5/3
  Divide3/1 -> e^3/1
  9/1 -> sqr9/1
  Product8/1 -> Subtract6/4
  Product7/1 -> Subtract6/3
  W4/1 -> Product8/2
  c2/1 -> Subtract2/2
  Product4/1 -> Divide4/2
  10/1 -> Product4/1
  e^3/1 -> Product5/1
  sqr6/1 -> Gain3/1
  6/1 -> Product2/1
  sqr3/1 -> Product1/2
  e^2/1 -> Product8/1
  Divide2/1 -> e^2/1
  Subtract2/1 -> sqr4/1
  Subtract6/1 -> Out1/1
  8/1 -> Product3/1
  sqr7/1 -> Product3/2
  Divide/1 -> e^/1
  5/1 -> sqr5/1
  3/1 -> sqr3/1
  4/1 -> Product1/1
  Gain2/1 -> Divide2/1
  Gain4/1 -> Divide4/1
  In1/1 -> Subtract5/1, Scope1/1
  W1/1 -> Product5/2
  sqr4/1 -> Gain2/1
  c3/1 -> Subtract3/2
  e^4/1 -> Product9/1
  sqr5/1 -> Product2/2
  sqr8/1 -> Gain4/1
  1/1 -> sqr1/1
  2/1 -> Product/1
  Product5/1 -> Subtract6/1
  Divide4/1 -> e^4/1
  W5/1 -> Product9/2
  7/1 -> sqr7/1
  Subtract/1 -> sqr/1
  Subtract5/1 -> Subtract2/1, Subtract4/1, Subtract3/1, Subtract/1, Subtract1/1, Display/1, Scope/1
  c1/1 -> Subtract1/2
  Subtract1/1 -> sqr2/1
  e^1/1 -> Product7/1
  Product9/1 -> Subtract6/5
  c4/1 -> Subtract4/2
  Subtract3/1 -> sqr6/1
  e^/1 -> Product6/1
  Product3/1 -> Divide3/2
  W2/1 -> Product6/2
  W3/1 -> Product7/2
  Gain1/1 -> Divide1/1
  Product6/1 -> Subtract6/2
  Product2/1 -> Divide2/2
  Gain/1 -> Divide/1
  Subtract4/1 -> sqr8/1
  Divide1/1 -> e^1/1
  Gain3/1 -> Divide3/1
  In2/1 -> Scope1/2, Subtract5/2
  sqr1/1 -> Product/2
  sqr2/1 -> Gain1/1
  Product/1 -> Divide/2
  sqr/1 -> Gain/1
  Product1/1 -> Divide1/2
  sqr9/1 -> Product4/2
  c/1 -> Subtract/2

== system singlcontact_control_smc_lqr_mydimes_reaction/Walking Robot/smc+lqr+neuro1+reaction1/SMC Controllers FL/Subsystem1 ==
  In1 : Inport
  In2 : Inport  Port=2
  {1,3,5,7,9} (5 alike) : Constant  Value=0.5
  {2,4,6,8,10} (5 alike) : Constant  Value=2
  Constant : Constant  Value=0
  Display : Display
  Divide{,1..4} (5 alike) : Product  Inputs=*/
  Gain{,1..4} (5 alike) : Gain  Gain=-1
  Product{,1..9} (10 alike) : Product
  Scope : Scope
  Scope1 : Scope  NumInputPorts=2
  Subtract{,1..4} (5 alike) : Sum  Inputs=+-
  Subtract5 : Sum  Inputs=+-+
  Subtract6 : Sum  Inputs=+++++
  W1 : Constant  Value=20
  W2 : Constant  Value=10
  W3 : Constant  Value=0
  W4 : Constant  Value=10
  W5 : Constant  Value=20
  c : Constant
  c1 : Constant  Value=0
  c2 : Constant  Value=-1
  c3 : Constant  Value=2
  c4 : Constant  Value=-2
  e^{,1..4} (5 alike) : Math
  sqr{,1..9} (10 alike) : Math  Operator=square
  Out1 : Outport
  wires:
  c/1 -> Subtract/2
  sqr9/1 -> Product4/2
  Product1/1 -> Divide1/2
  sqr/1 -> Gain/1
  Product/1 -> Divide/2
  sqr2/1 -> Gain1/1
  sqr1/1 -> Product/2
  In2/1 -> Subtract5/2, Scope1/2
  Gain3/1 -> Divide3/1
  Divide1/1 -> e^1/1
  Subtract4/1 -> sqr8/1
  Gain/1 -> Divide/1
  Product2/1 -> Divide2/2
  Product6/1 -> Subtract6/2
  Gain1/1 -> Divide1/1
  W3/1 -> Product7/2
  W2/1 -> Product6/2
  Product3/1 -> Divide3/2
  e^/1 -> Product6/1
  Subtract3/1 -> sqr6/1
  c4/1 -> Subtract4/2
  Product9/1 -> Subtract6/5
  e^1/1 -> Product7/1
  Subtract1/1 -> sqr2/1
  c1/1 -> Subtract1/2
  Subtract5/1 -> Scope/1, Display/1, Subtract1/1, Subtract/1, Subtract3/1, Subtract4/1, Subtract2/1
  Subtract/1 -> sqr/1
  7/1 -> sqr7/1
  W5/1 -> Product9/2
  Divide4/1 -> e^4/1
  Product5/1 -> Subtract6/1
  2/1 -> Product/1
  1/1 -> sqr1/1
  sqr8/1 -> Gain4/1
  sqr5/1 -> Product2/2
  e^4/1 -> Product9/1
  c3/1 -> Subtract3/2
  sqr4/1 -> Gain2/1
  W1/1 -> Product5/2
  In1/1 -> Scope1/1, Subtract5/1
  Gain4/1 -> Divide4/1
  Gain2/1 -> Divide2/1
  4/1 -> Product1/1
  3/1 -> sqr3/1
  5/1 -> sqr5/1
  Divide/1 -> e^/1
  sqr7/1 -> Product3/2
  8/1 -> Product3/1
  Subtract6/1 -> Out1/1
  Subtract2/1 -> sqr4/1
  Divide2/1 -> e^2/1
  e^2/1 -> Product8/1
  sqr3/1 -> Product1/2
  6/1 -> Product2/1
  sqr6/1 -> Gain3/1
  e^3/1 -> Product5/1
  10/1 -> Product4/1
  Product4/1 -> Divide4/2
  c2/1 -> Subtract2/2
  W4/1 -> Product8/2
  Product7/1 -> Subtract6/3
  Product8/1 -> Subtract6/4
  9/1 -> sqr9/1
  Divide3/1 -> e^3/1
  Constant/1 -> Subtract5/3

== system singlcontact_control_smc_lqr_mydimes_reaction/Walking Robot/smc+lqr+neuro1+reaction1/SMC Controllers FL/Subsystem2 ==
  <knee_angle> : Inport
  <hip_pitch_angle> : Inport  Port=2
  Gain3 : Gain  Gain=0.5
  Product : Product
  Product3 : Product
  length from ground : Subsystem
  Input : Outport
  Input1 : Outport  Port=2
  wires:
  Product/1 -> Input/1
  length from ground/2(Outport) -> Product3/1
  Gain3/1 -> Product/2, Product3/2
  Product3/1 -> Input1/1
  [Rfl] -> Gain3/1
  <hip_pitch_angle>/1 -> length from ground/2(In2)
  <knee_angle>/1 -> length from ground/1(In1)
  length from ground/1(Output) -> Product/1

== system singlcontact_control_smc_lqr_mydimes_reaction/Walking Robot/smc+lqr+neuro1+reaction1/SMC Controllers FR/Equivalent control ==
  theta2 : Inport
  theta1 : Inport  Port=2
  theta2ddot : Inport  Port=3
  theta1dot : Inport  Port=4
  theta2dot : Inport  Port=5
  theta1ddot : Inport  Port=6
  theta3 : Inport  Port=7
  theta4 : Inport  Port=8
  theta1dot1 : Inport  Port=9
  Constant : Constant  Value=0
  Constant1 : Constant  Value=0
  SMC equivalent T1 : Subsystem
  SMC equivalent T2 : Subsystem
  Scope : Scope  NumInputPorts=2
  tag scope: TT1FR=global, TT2FR=global
  wires:
  SMC equivalent T2/1(T2) -> Scope/1, [TT2FR]
  theta2/1 -> SMC equivalent T1/1(theta2)
  SMC equivalent T1/1(T1) -> Scope/2, [TT1FR]
  Constant1/1 -> SMC equivalent T2/4(theta2ddot)
  theta2ddot/1 -> SMC equivalent T1/3(theta2ddot)
  theta1dot/1 -> SMC equivalent T1/4(theta1dot)
  Constant/1 -> SMC equivalent T1/6(theta1ddot)
  theta3/1 -> SMC equivalent T2/2(theta2)
  theta1/1 -> SMC equivalent T1/2(theta1)
  theta4/1 -> SMC equivalent T2/3(theta1)
  theta1ddot/1 -> SMC equivalent T2/1(theta1ddot)
  theta2dot/1 -> SMC equivalent T1/5(theta2dot)
  theta1dot1/1 -> SMC equivalent T2/5(theta1dot)

== system singlcontact_control_smc_lqr_mydimes_reaction/Walking Robot/smc+lqr+neuro1+reaction1/SMC Controllers FR/SMC ==
  In1 : Inport
  In2 : Inport  Port=2
  T1_neuro : Inport  Port=3
  T2_neuro : Inport  Port=4
  Input : Inport  Port=5
  Input1 : Inport  Port=6
  Edot : Derivative
  Edot1 : Derivative
  Gain : Gain  Gain=-0.85
  Gain1 : Gain  Gain=-0.7
  Mux : Mux  Inputs=2
  New : Gain  Gain=knee_smc_new
  New1 : Gain  Gain=hip_smc_new
  Product : Product
  Product2 : Product
  Random Source : dspobslib/Random Source  SrcType=Uniform  NormMethod=Ziggurat  CltLength=12  MinVal=-4  MaxVal=4  MeanVal=0  VarVal=1  RepMode=Not repeatable  rawSeed=1  IsInherit=off  SampMode=Discrete  SampTime=0.05  SampFrame=1  DataType=Double  OutComplex=Real  OutputFrames=off
  Random Source1 : dspobslib/Random Source  SrcType=Uniform  NormMethod=Ziggurat  CltLength=12  MinVal=-4  MaxVal=4  MeanVal=0  VarVal=1  RepMode=Not repeatable  rawSeed=1  IsInherit=off  SampMode=Discrete  SampTime=0.05  SampFrame=1  DataType=Double  OutComplex=Real  OutputFrames=off
  S : Sum
  S1 : Sum
  Scope{2..5} (4 alike) : Scope
  Sum : Sum  Inputs=+++++
  Sum1 : Sum  Inputs=+++++
  Tanh : Trigonometry  Operator=tanh
  Tanh1 : Trigonometry  Operator=tanh
  lamda : Constant  Value=knee_smc_lamda
  lamda1 : Constant  Value=hip_smc_lamda
  Out1 : Outport
  tag scope: edotFR1=global, edotFR2=global, lamdaFR1=global, lamdaFR2=global, slFR1=global, slFR2=global
  wires:
  S1/1 -> [slFR2], Tanh/1
  Edot/1 -> [edotFR1], S/1
  Product/1 -> S/2
  lamda1/1 -> [lamdaFR2], Product2/1
  In2/1 -> Product2/2, Edot1/1
  Product2/1 -> S1/2
  In1/1 -> Edot/1, Product/2
  Edot1/1 -> S1/1, [edotFR2]
  Tanh1/1 -> New/1
  lamda/1 -> [lamdaFR1], Product/1
  Tanh/1 -> New1/1
  [TT1FR] -> Sum/2
  [TT2FR] -> Sum1/2
  Mux/1 -> Out1/1
  Sum/1 -> Scope3/1, Scope5/1, Mux/1
  Sum1/1 -> Scope4/1, Mux/2, Scope2/1
  T1_neuro/1 -> Sum/3
  T2_neuro/1 -> Sum1/3
  S/1 -> [slFR1], Tanh1/1
  New/1 -> Gain/1, Sum/1
  Gain/1 -> Sum/4
  Gain1/1 -> Sum1/4
  New1/1 -> Sum1/1, Gain1/1
  Random Source/1 -> ?
  Random Source1/1 -> ?
  Input/1 -> Sum/5
  Input1/1 -> Sum1/5

== system singlcontact_control_smc_lqr_mydimes_reaction/Walking Robot/smc+lqr+neuro1+reaction1/SMC Controllers FR/Subsystem ==
  In1 : Inport
  In2 : Inport  Port=2
  {1,3,5,7,9} (5 alike) : Constant  Value=0.5
  {2,4,6,8,10} (5 alike) : Constant  Value=2
  Constant : Constant  Value=0
  Display : Display
  Divide{,1..4} (5 alike) : Product  Inputs=*/
  Gain{,1..4} (5 alike) : Gain  Gain=-1
  Product{,1..9} (10 alike) : Product
  Scope : Scope
  Scope1 : Scope  NumInputPorts=2
  Subtract{,1..4} (5 alike) : Sum  Inputs=+-
  Subtract5 : Sum  Inputs=+-+
  Subtract6 : Sum  Inputs=+++++
  W1 : Constant  Value=30
  W2 : Constant  Value=15
  W3 : Constant  Value=0
  W4 : Constant  Value=15
  W5 : Constant  Value=30
  c : Constant
  c1 : Constant  Value=0
  c2 : Constant  Value=-1
  c3 : Constant  Value=2
  c4 : Constant  Value=-2
  e^{,1..4} (5 alike) : Math
  sqr{,1..9} (10 alike) : Math  Operator=square
  Out1 : Outport
  wires:
  c/1 -> Subtract/2
  sqr9/1 -> Product4/2
  Product1/1 -> Divide1/2
  sqr/1 -> Gain/1
  Product/1 -> Divide/2
  sqr2/1 -> Gain1/1
  sqr1/1 -> Product/2
  In2/1 -> Subtract5/2, Scope1/2
  Gain3/1 -> Divide3/1
  Divide1/1 -> e^1/1
  Subtract4/1 -> sqr8/1
  Gain/1 -> Divide/1
  Product2/1 -> Divide2/2
  Product6/1 -> Subtract6/2
  Gain1/1 -> Divide1/1
  W3/1 -> Product7/2
  W2/1 -> Product6/2
  Product3/1 -> Divide3/2
  e^/1 -> Product6/1
  Subtract3/1 -> sqr6/1
  c4/1 -> Subtract4/2
  Product9/1 -> Subtract6/5
  e^1/1 -> Product7/1
  Subtract1/1 -> sqr2/1
  c1/1 -> Subtract1/2
  Subtract5/1 -> Scope/1, Display/1, Subtract1/1, Subtract/1, Subtract3/1, Subtract4/1, Subtract2/1
  Subtract/1 -> sqr/1
  7/1 -> sqr7/1
  W5/1 -> Product9/2
  Divide4/1 -> e^4/1
  Product5/1 -> Subtract6/1
  2/1 -> Product/1
  1/1 -> sqr1/1
  sqr8/1 -> Gain4/1
  sqr5/1 -> Product2/2
  e^4/1 -> Product9/1
  c3/1 -> Subtract3/2
  sqr4/1 -> Gain2/1
  W1/1 -> Product5/2
  In1/1 -> Scope1/1, Subtract5/1
  Gain4/1 -> Divide4/1
  Gain2/1 -> Divide2/1
  4/1 -> Product1/1
  3/1 -> sqr3/1
  5/1 -> sqr5/1
  Divide/1 -> e^/1
  sqr7/1 -> Product3/2
  8/1 -> Product3/1
  Subtract6/1 -> Out1/1
  Subtract2/1 -> sqr4/1
  Divide2/1 -> e^2/1
  e^2/1 -> Product8/1
  sqr3/1 -> Product1/2
  6/1 -> Product2/1
  sqr6/1 -> Gain3/1
  e^3/1 -> Product5/1
  10/1 -> Product4/1
  Product4/1 -> Divide4/2
  c2/1 -> Subtract2/2
  W4/1 -> Product8/2
  Product7/1 -> Subtract6/3
  Product8/1 -> Subtract6/4
  9/1 -> sqr9/1
  Divide3/1 -> e^3/1
  Constant/1 -> Subtract5/3
